simulink model "Modelo_cinematico_directo_central"  (R2016a)
settings: Solver=FixedStepAuto  StartTime=0.0  StopTime=10.0  RelTol=1e-3
settings Model: Creator=daniel  LastModifiedBy=daniel
settings HardwareCC: ProdBitPerPointer=32  ProdWordSize=32  ProdHWDeviceType=Intel->x86-32 (Windows32)

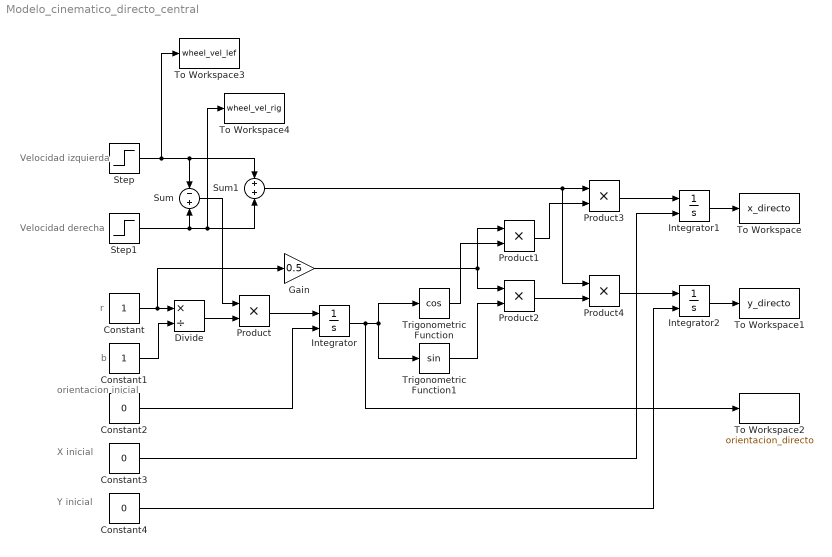
== system Modelo_cinematico_directo_central ==
  note: orientacion
      | inicial
  note: b
  note: r
  note: Velocidad izquierda
  note: Velocidad derecha
  note: X
      | inicial
  note: Y
      | inicial
  Constant : Constant
  Constant1 : Constant
  Constant2 : Constant  Value=0
  Constant3 : Constant  Value=0
  Constant4 : Constant  Value=0
  Divide : Product  Inputs=*/
  Gain : Gain  Gain=0.5
  Integrator : Integrator  InitialConditionSource=external
  Integrator1 : Integrator  InitialConditionSource=external
  Integrator2 : Integrator  InitialConditionSource=external
  Product{,1..4} (5 alike) : Product
  Step : Step  SampleTime=0
  Step1 : Step  Time=5  SampleTime=0
  Sum : Sum  Inputs=-+
  Sum1 : Sum
  To Workspace : ToWorkspace  VariableName=x_directo  SaveFormat=Timeseries  SampleTime=-1
  To Workspace1 : ToWorkspace  VariableName=y_directo  SaveFormat=Timeseries  SampleTime=-1
  To Workspace2 : ToWorkspace  VariableName=orientacion_directo  SaveFormat=Timeseries  SampleTime=-1
  To Workspace3 : ToWorkspace  VariableName=wheel_vel_lef  SaveFormat=Timeseries  SampleTime=-1
  To Workspace4 : ToWorkspace  VariableName=wheel_vel_rig  SaveFormat=Timeseries  SampleTime=-1
  Trigonometric Function : Trigonometry  Operator=cos  OutputSignalType=real
  Trigonometric Function1 : Trigonometry  OutputSignalType=real
  wires:
  Constant/1 -> Gain/1, Divide/1
  Constant1/1 -> Divide/2
  Divide/1 -> Product/2
  Sum/1 -> Product/1
  Product/1 -> Integrator/1
  Constant2/1 -> Integrator/2
  Integrator/1 -> To Workspace2/1, Trigonometric Function1/1, Trigonometric Function/1
  Trigonometric Function1/1 -> Product2/2
  Trigonometric Function/1 -> Product1/2
  Gain/1 -> Product1/1, Product2/1
  Sum1/1 -> Product3/1, Product4/1
  Product1/1 -> Product3/2
  Product2/1 -> Product4/2
  Product4/1 -> Integrator2/1
  Product3/1 -> Integrator1/1
  Integrator2/1 -> To Workspace1/1
  Integrator1/1 -> To Workspace/1
  Constant3/1 -> Integrator1/2
  Constant4/1 -> Integrator2/2
  Step1/1 -> To Workspace4/1, Sum1/2, Sum/2
  Step/1 -> To Workspace3/1, Sum1/1, Sum/1
